simulink model "Valve_TestBed"  (R2015a)
settings: Solver=FixedStepDiscrete  StartTime=0.0  StopTime=1  FixedStep=1  RelTol=1e-3
undefined symbols (not defined in the file): MWS
libraries: Lib_Turbo_Valve_TMATS x1
settings Model: Creator=jwchapm2  LastModifiedBy=jwchapm2
settings OptimizationCC: ExpressionDepthLimit=2147483647
settings DebuggingCC: UnderspecifiedInitializationDetection=Classic  MergeDetectMultiDrivingBlocksExec=none  SolverPrmCheckMsg=warning  StateNameClashWarn=warning

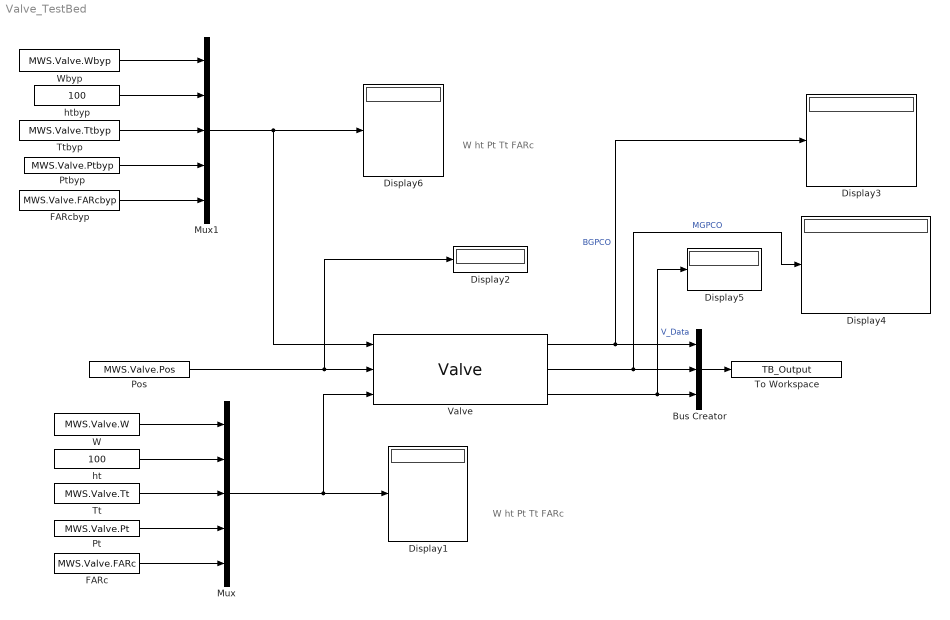
== system Valve_TestBed ==
  note: W
      | ht
      | Pt
      | Tt
      | FARc
  note: W
      | ht
      | Pt
      | Tt
      | FARc
  Bus Creator : BusCreator  Inputs=3
  Display{1..6} (6 alike) : Display
  FARc : Constant  Value=MWS.Valve.FARc
  FARcbyp : Constant  Value=MWS.Valve.FARcbyp
  Mux : Mux  Inputs=5
  Mux1 : Mux  Inputs=5
  Pos : Constant  Value=MWS.Valve.Pos
  Pt : Constant  Value=MWS.Valve.Pt
  Ptbyp : Constant  Value=MWS.Valve.Ptbyp
  To Workspace : ToWorkspace  VariableName=TB_Output  SampleTime=-1
  Tt : Constant  Value=MWS.Valve.Tt
  Ttbyp : Constant  Value=MWS.Valve.Ttbyp
  Valve : Lib_Turbo_Valve_TMATS/Valve  VFO_M=MWS.Valve.VFO  VDZ_M=MWS.Valve.VDZ  VAe_M=MWS.Valve.VAA  X_VPRVec_M=MWS.Valve.PRvec  T_VWArray_M=MWS.Valve.VWArray
  W : Constant  Value=MWS.Valve.W
  Wbyp : Constant  Value=MWS.Valve.Wbyp
  ht : Constant  Value=100
  htbyp : Constant  Value=100
  wires:
  Pos/1 -> Display2/1, Valve/2
  W/1 -> Mux/1
  FARc/1 -> Mux/5
  Tt/1 -> Mux/3
  Pt/1 -> Mux/4
  Mux/1 -> Valve/3, Display1/1
  Valve/1 -> Display3/1, Bus Creator/1  "BGPCO"
  Valve/2 -> Display4/1, Bus Creator/2  "MGPCO"
  Valve/3 -> Display5/1, Bus Creator/3  "V_Data"
  Bus Creator/1 -> To Workspace/1
  ht/1 -> Mux/2
  Wbyp/1 -> Mux1/1
  FARcbyp/1 -> Mux1/5
  Ttbyp/1 -> Mux1/3
  Ptbyp/1 -> Mux1/4
  Mux1/1 -> Valve/1, Display6/1
  htbyp/1 -> Mux1/2
